simulink model "Assignment3_2019"  (R2019a)
settings: Solver=VariableStepAuto  StartTime=0.0  StopTime=30  RelTol=1e-3
model workspace (MAT data in the model file):
  A = 1
  Cd = 0.01
  Cr = 1e-07
  I = 10
  KD = 0
  KI = 8
  KP = 500
  MD = 2
  Rho = 0.1
  T = 400
  Vr = 20
  alpha_n = 0.002
  d = 10
  g = 9.81
  m = 1200
  sin_zheta = 0
settings Model: OrderedModelArguments=off  Creator=Pongsakorn  LastModifiedBy=Pongsakorn

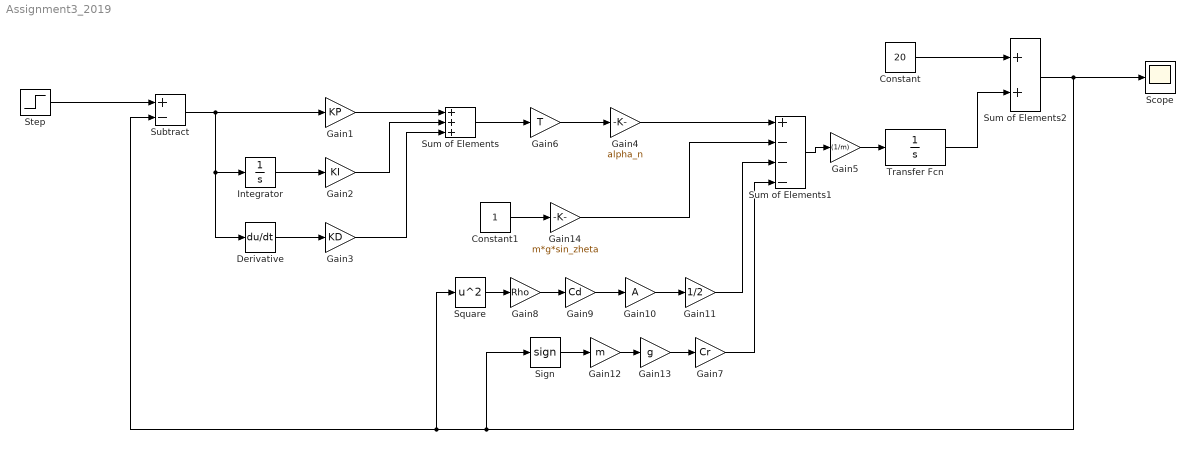
== system Assignment3_2019 ==
  Constant : Constant  Value=20
  Constant1 : Constant
  Derivative : Derivative
  Gain1 : Gain  Gain=KP
  Gain10 : Gain  Gain=A
  Gain11 : Gain  Gain=1/2
  Gain12 : Gain  Gain=m
  Gain13 : Gain  Gain=g
  Gain14 : Gain  Gain=m*g*sin_zheta
  Gain2 : Gain  Gain=KI
  Gain3 : Gain  Gain=KD
  Gain4 : Gain  Gain=alpha_n
  Gain5 : Gain  Gain=(1/m)
  Gain6 : Gain  Gain=T
  Gain7 : Gain  Gain=Cr
  Gain8 : Gain  Gain=Rho
  Gain9 : Gain  Gain=Cd
  Integrator : Integrator
  Scope : Scope
  Sign : Signum  ZeroCross=off
  Square : Math  Operator=square  SaturateOnIntegerOverflow=on
  Step : Step  After=Vr  SampleTime=0
  Subtract : Sum  Inputs=+-
  Sum of Elements : Sum  Inputs=+++  CollapseMode=Specified dimension  CollapseDim=3
  Sum of Elements1 : Sum  Inputs=+---  CollapseMode=Specified dimension  CollapseDim=3
  Sum of Elements2 : Sum  CollapseMode=Specified dimension  CollapseDim=3
  Transfer Fcn : TransferFcn  Denominator=[1 0]
  wires:
  Subtract/1 -> Derivative/1, Integrator/1, Gain1/1
  Integrator/1 -> Gain2/1
  Derivative/1 -> Gain3/1
  Gain1/1 -> Sum of Elements/1
  Sum of Elements1/1 -> Gain5/1
  Sum of Elements/1 -> Gain6/1
  Sign/1 -> Gain12/1
  Square/1 -> Gain8/1
  Gain6/1 -> Gain4/1
  Gain5/1 -> Transfer Fcn/1
  Gain8/1 -> Gain9/1
  Gain2/1 -> Sum of Elements/2
  Gain3/1 -> Sum of Elements/3
  Step/1 -> Subtract/1
  Gain9/1 -> Gain10/1
  Gain10/1 -> Gain11/1
  Gain12/1 -> Gain13/1
  Gain13/1 -> Gain7/1
  Constant/1 -> Sum of Elements2/1
  Transfer Fcn/1 -> Sum of Elements2/2
  Sum of Elements2/1 -> Sign/1, Square/1, Subtract/2, Scope/1
  Gain4/1 -> Sum of Elements1/1
  Gain11/1 -> Sum of Elements1/3
  Constant1/1 -> Gain14/1
  Gain7/1 -> Sum of Elements1/4
  Gain14/1 -> Sum of Elements1/2
